simulink model "TrayectoriasTiempoIgual"  (R2021b)
settings: Solver=VariableStepAuto  StartTime=0.0  StopTime=50  RelTol=1e-3
settings Model: Creator=fabia  LastModifiedBy=fabia

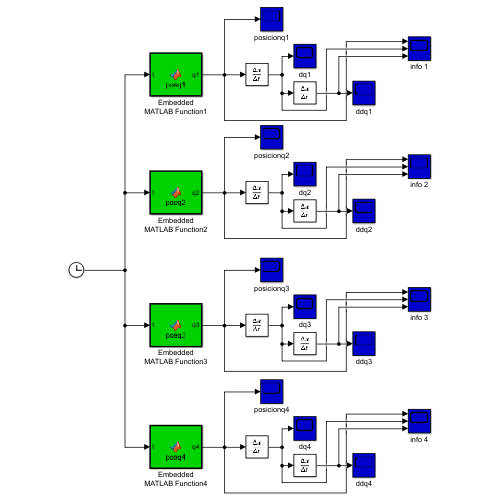
[thumbnail: Simulink's stored preview of the top-level diagram]
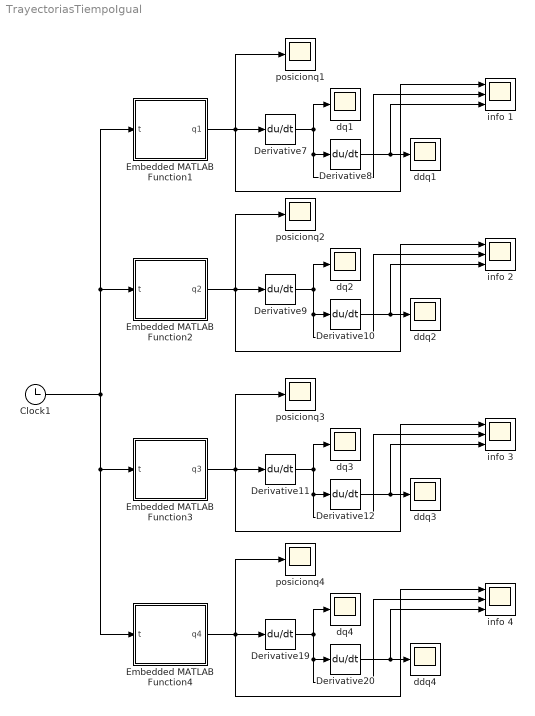
== system TrayectoriasTiempoIgual ==
  Clock1 : Clock
      settings: Decimation=1000
  Derivative{7..12,19..20} (8 alike) : Derivative
  Embedded MATLAB Function1 : MATLAB Function  TreatAsAtomicUnit=on
  Embedded MATLAB Function2 : MATLAB Function  TreatAsAtomicUnit=on
  Embedded MATLAB Function3 : MATLAB Function  TreatAsAtomicUnit=on
  Embedded MATLAB Function4 : MATLAB Function  TreatAsAtomicUnit=on
  ddq{1..4} (4 alike) : Scope
  dq{1..4} (4 alike) : Scope
  info {1..4} (4 alike) : Scope  NumInputPorts=3
  posicionq{1..4} (4 alike) : Scope
  wires:
  Embedded MATLAB Function2/1(q2) -> info 2/1, posicionq2/1, Derivative9/1
  Derivative11/1 -> info 3/2, Derivative12/1, dq3/1
  Derivative8/1 -> info 1/3, ddq1/1
  Derivative7/1 -> info 1/2, Derivative8/1, dq1/1
  Embedded MATLAB Function3/1(q3) -> info 3/1, posicionq3/1, Derivative11/1
  Derivative20/1 -> info 4/3, ddq4/1
  Clock1/1 -> Embedded MATLAB Function2/1(t), Embedded MATLAB Function1/1(t), Embedded MATLAB Function4/1(t), Embedded MATLAB Function3/1(t)
  Embedded MATLAB Function1/1(q1) -> info 1/1, posicionq1/1, Derivative7/1
  Embedded MATLAB Function4/1(q4) -> info 4/1, posicionq4/1, Derivative19/1
  Derivative19/1 -> info 4/2, Derivative20/1, dq4/1
  Derivative9/1 -> info 2/2, Derivative10/1, dq2/1
  Derivative10/1 -> info 2/3, ddq2/1
  Derivative12/1 -> info 3/3, ddq3/1

== matlab function TrayectoriasTiempoIgual/Embedded MATLAB Function2 ==
  data: q2 output; t input
function q2 = posq2(t)
% This block supports an embeddable subset of the MATLAB language.
% See the help menu for details. 

if (t>=17)  % Si el t>=tmax, se repite una vez la rutina
    t=t-17;
end

if(t<6) % Movimiento 1
    t_inic = 0; % Tiempo en que inicia
    tf = 4;     % Tiempo en que termina
    y_ini = 0.785;
    y_f = -1.570;
elseif (t>=6 && t<12) % Movimiento 2
    t_inic = 6;
    tf = 4;
    y_ini =  -1.5706;
    y_f =  -1.570;
else  % Movimiento 3
    t_inic = 12;
    tf = 5;
    y_ini =  -1.570;
    y_f = 0.785;
end

% Calculo de trayectoria de tiempo minimo
Tb = tf/2;
% Vmax = 2*(y_f - y_ini)/(tf);
Vmax = (y_f - y_ini)/(tf - Tb);
ta = t - t_inic;
if(ta<0)
    q2 = y_ini;
elseif(ta >= 0 && ta < Tb)
    q2 = y_ini + (Vmax/(2*Tb))*ta*ta;
elseif(ta >= Tb && ta < (tf - Tb))
    q2 = (y_ini + y_f - Vmax*tf)/2 + Vmax*ta;
elseif(ta >= (tf - Tb) && ta < tf)
     q2 = y_f - (Vmax*(tf-ta)*(tf-ta)/(2*Tb));
else
    q2 = y_f;
end

== matlab function TrayectoriasTiempoIgual/Embedded MATLAB Function3 ==
  data: q3 output; t input
function q3 = posq3(t)
% This block supports an embeddable subset of the MATLAB language.
% See the help menu for details. 

if (t>=17)  % Si el t>=tmax, se repite una vez la rutina
    t=t-17;
end

if(t<6) % Movimiento 1
    t_inic = 0; % Tiempo en que inicia
    tf = 4;     % Tiempo en que termina
    y_ini = 1.570;
    y_f = -0.785;
elseif (t>=6 && t<12) % Movimiento 2
    t_inic = 6;
    tf = 4;
    y_ini = -0.785;
    y_f = -0.785;
else  % Movimiento 3
    t_inic = 12;
    tf = 5;
    y_ini = -0.785;
    y_f =  1.570;
end

% Calculo de trayectoria de tiempo minimo
Tb = tf/2;
% Vmax = 2*(y_f - y_ini)/(tf);
Vmax = (y_f - y_ini)/(tf - Tb);
ta = t - t_inic;
if(ta<0)
    q3 = y_ini;
elseif(ta >= 0 && ta < Tb)
    q3 = y_ini + (Vmax/(2*Tb))*ta*ta;
elseif(ta >= Tb && ta < (tf - Tb))
    q3 = (y_ini + y_f - Vmax*tf)/2 + Vmax*ta;
elseif(ta >= (tf - Tb) && ta < tf)
     q3 = y_f - (Vmax*(tf-ta)*(tf-ta)/(2*Tb));
else
    q3 = y_f;
end

== matlab function TrayectoriasTiempoIgual/Embedded MATLAB Function4 ==
  data: q4 output; t input
function q4 = posq4(t)
% This block supports an embeddable subset of the MATLAB language.
% See the help menu for details. 

if (t>=17)  % Si el t>=tmax, se repite una vez la rutina
    t=t-17;
end

if(t<6) % Movimiento 1
    t_inic = 0; % Tiempo en que inicia
    tf = 4;     % Tiempo en que termina
    y_ini = 3.14159;
    y_f = 0;
elseif (t>=6 && t<12) % Movimiento 2
    t_inic = 6;
    tf = 4;
    y_ini = 0;
    y_f = 0;
else  % Movimiento 3
    t_inic = 12;
    tf = 5;
    y_ini = 0;
    y_f = 3.14159;
end

% Calculo de trayectoria de tiempo minimo
Tb = tf/2;
% Vmax = 2*(y_f - y_ini)/(tf);
Vmax = (y_f - y_ini)/(tf - Tb);
ta = t - t_inic;
if(ta<0)
    q4 = y_ini;
elseif(ta >= 0 && ta < Tb)
    q4 = y_ini + (Vmax/(2*Tb))*ta*ta;
elseif(ta >= Tb && ta < (tf - Tb))
    q4 = (y_ini + y_f - Vmax*tf)/2 + Vmax*ta;
elseif(ta >= (tf - Tb) && ta < tf)
     q4 = y_f - (Vmax*(tf-ta)*(tf-ta)/(2*Tb));
else
    q4 = y_f;
end

== matlab function TrayectoriasTiempoIgual/Embedded MATLAB Function1 ==
  data: q1 output; t input
function q1 = posq1(t)
% This block supports an embeddable subset of the MATLAB language.
% See the help menu for details. 

if (t>=17)  % Si el t>=tmax, se repite otra vez la rutina
    t=t-17;
end

if(t<6) % Movimiento 1
    t_inic = 0; % Tiempo en que inicia
    tf = 4;     % Tiempo en que termina
    y_ini = 0;  % Posicion articular inicial (rad)
    y_f = -3.14159;    % Posicion articular final (rad)
elseif (t>=6 && t<12) % Movimiento 2
    t_inic = 6;
    tf = 4;
    y_ini = -3.14159;
    y_f =-3.14159;
else  % Movimiento 3
    t_inic = 12;
    tf = 5;
    y_ini =-3.14159;
    y_f = 0;
end

% Calculo de trayectoria de tiempo minimo
Tb = tf/2;  % el tb queda a la mitad del tiempo final

% Vmax = 2*(y_f - y_ini)/(tf);

Vmax = (y_f - y_ini)/(tf - Tb);
ta = t - t_inic;

% Polinomios que describen la curva en funcion de tiempo
if(ta<0)
    q1 = y_ini;
elseif(ta >= 0 && ta < Tb)
    q1 = y_ini + (Vmax/(2*Tb))*ta*ta;
elseif(ta >= Tb && ta < (tf - Tb))
    q1 = (y_ini + y_f - Vmax*tf)/2 + Vmax*ta;
elseif(ta >= (tf - Tb) && ta < tf)
     q1 = y_f - (Vmax*(tf-ta)*(tf-ta)/(2*Tb));
else
    q1 = y_f;
end
